simulink model "EngineModel_scaled_27_7_2016_with_new_maps"  (R2021a)
settings: Solver=ode4  StartTime=0.0  StopTime=30  FixedStep=0.2  RelTol=1e-3  EnableMultiTasking=on
values from neighbouring files (symbols this model uses):
  Fanmap_2 = [1 1 1 1 1 1 1 1 1 1 275.724 325.4224 ... (330 elements, 10x3x11)]    [enginemaps2.mat]
  HPCompmap_2 = [1 1 1 1 1 1 1 1 1 1 32.390865 37.6623195 ... (330 elements, 10x3x11)]    [enginemaps2.mat]
  HPTurbinemap_2 = [0.24979968 0.24979968 0.24979968 0.24979968 0.24979968 0.24979968 0.24979968 0.24979968 0.24979968 0.24979968 0.004250667 0.005047667 ... (330 elements, 10x3x11)]    [enginemaps2.mat]
  LPCompmap_2 = [1 1 1 1 1 1 1 1 1 1 34.17260994 40.23277722 ... (330 elements, 10x3x11)]    [enginemaps2.mat]
  LPTurbinemap_2 = [0.665969797 0.665969797 0.665969797 0.665969797 0.665969797 0.665969797 0.665969797 0.665969797 0.00912 0.013173333 0.015706667 0.01672 ... (264 elements, 8x3x11)]    [enginemaps2.mat]
undefined symbols (not defined in the file or in its folder): Adiabatic_compression_fan, Adiabatic_compression_HPC, Adiabatic_compression_LPC, coldnozzle, compression_ram, cond_f2, D, datatables, hotnozzle, HPT1, if_Nth, if_Ntl, if_Z, LPT, performance1, thermo_combustor, turbo
libraries: dspmtrx3 x10, aerolibatmos2 x8, dspsigattribs x3, dspsolvers x2, dspfactors x1
(part 14 of 14)

== system EngineModel_scaled_27_7_2016_with_new_maps/Double spool TFE CF6-50 steady state modeling (BOING 747-200)/Error Due to Vs/Error Due To Dv7/HPT/enthalpy_MAPS/HPT map/HPT Map lookup Table Efficency/if_Nth ==
  TFth : Inport
  Nth : Inport  Port=2
  Demux : Demux  Outputs=1
      settings: DisplayOption=none
  Interpreted MATLAB Function : MATLABFcn  MATLABFcn=if_Nth(u(1),u(2))  OutputDimensions=1
  Mux : Mux  Inputs=2
      settings: DisplayOption=signals
  Zthi : Outport
  wires:
  Interpreted MATLAB Function/1 -> Demux/1
  TFth/1 -> Mux/1
  Mux/1 -> Interpreted MATLAB Function/1
  Demux/1 -> Zthi/1
  Nth/1 -> Mux/2

== system EngineModel_scaled_27_7_2016_with_new_maps/Double spool TFE CF6-50 steady state modeling (BOING 747-200)/Error Due to Vs/Error Due To Dv7/LPT/enthalpy_MAPS/LPT map/LPT Map lookup Table (DH//T)/If condition Ztl ==
  Ztli : Inport
  Demux : Demux  Outputs=1
      settings: DisplayOption=none
  Interpreted MATLAB Function : MATLABFcn  MATLABFcn=if_Z(u(1))  OutputDimensions=1
  Mux : Mux  Inputs=1
      settings: DisplayOption=signals
  Ztl : Outport
  wires:
  Interpreted MATLAB Function/1 -> Demux/1
  Mux/1 -> Interpreted MATLAB Function/1
  Demux/1 -> Ztl/1
  Ztli/1 -> Mux/1

== system EngineModel_scaled_27_7_2016_with_new_maps/Double spool TFE CF6-50 steady state modeling (BOING 747-200)/Error Due to Vs/Error Due To Dv7/LPT/enthalpy_MAPS/LPT map/LPT Map lookup Table (DH//T)/if_Ntl ==
  TFtl : Inport
  Ntl : Inport  Port=2
  Demux : Demux  Outputs=1
      settings: DisplayOption=none
  Interpreted MATLAB Function : MATLABFcn  MATLABFcn=if_Ntl(u(1),u(2))  OutputDimensions=1
  Mux : Mux  Inputs=2
      settings: DisplayOption=signals
  Ztli : Outport
  wires:
  Interpreted MATLAB Function/1 -> Demux/1
  TFtl/1 -> Mux/1
  Mux/1 -> Interpreted MATLAB Function/1
  Demux/1 -> Ztli/1
  Ntl/1 -> Mux/2

== system EngineModel_scaled_27_7_2016_with_new_maps/Double spool TFE CF6-50 steady state modeling (BOING 747-200)/Error Due to Vs/Error Due To Dv7/LPT/enthalpy_MAPS/LPT map/LPT Map lookup Table Efficency/If condition Ztl ==
  Ztli : Inport
  Demux : Demux  Outputs=1
      settings: DisplayOption=none
  Interpreted MATLAB Function : MATLABFcn  MATLABFcn=if_Z(u(1))  OutputDimensions=1
  Mux : Mux  Inputs=1
      settings: DisplayOption=signals
  Ztl : Outport
  wires:
  Interpreted MATLAB Function/1 -> Demux/1
  Mux/1 -> Interpreted MATLAB Function/1
  Demux/1 -> Ztl/1
  Ztli/1 -> Mux/1

== system EngineModel_scaled_27_7_2016_with_new_maps/Double spool TFE CF6-50 steady state modeling (BOING 747-200)/Error Due to Vs/Error Due To Dv7/LPT/enthalpy_MAPS/LPT map/LPT Map lookup Table Efficency/if_Ntl ==
  TFtl : Inport
  Ntl : Inport  Port=2
  Demux : Demux  Outputs=1
      settings: DisplayOption=none
  Interpreted MATLAB Function : MATLABFcn  MATLABFcn=if_Ntl(u(1),u(2))  OutputDimensions=1
  Mux : Mux  Inputs=2
      settings: DisplayOption=signals
  Ztli : Outport
  wires:
  Interpreted MATLAB Function/1 -> Demux/1
  TFtl/1 -> Mux/1
  Mux/1 -> Interpreted MATLAB Function/1
  Demux/1 -> Ztli/1
  Ntl/1 -> Mux/2
